simulink model "sampleModel1865"  (R2023a)
settings: Solver=VariableStepAuto  StartTime=0.0  StopTime=10.0  RelTol=1e-3
libraries: simulink x2, hdlsllib x2
settings Model: Creator=user1  LastModifiedBy=user1

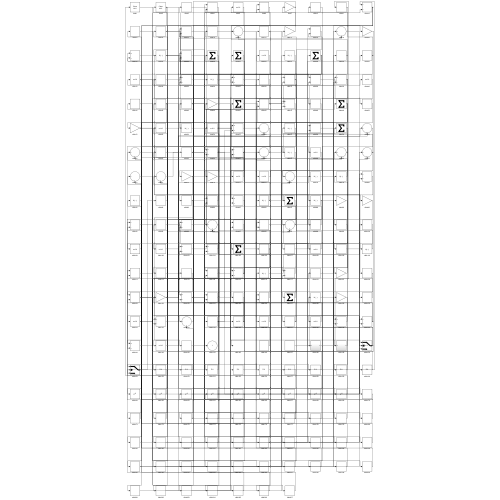
[thumbnail: Simulink's stored preview of the top-level diagram]
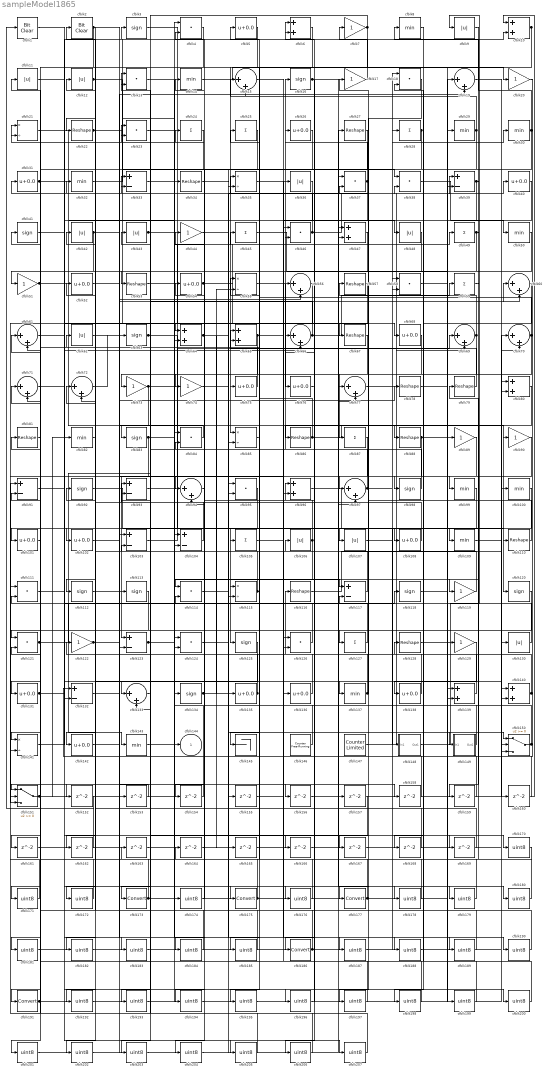
== system sampleModel1865 ==
  cfblk1 : simulink/Logic and Bit Operations/Bit Clear  iBit=0
      settings: LibrarySourceBlock=|
      | hdlsllib/Logic and Bit
      | Operations/Bit Clear
  cfblk{6,10,47,64..65,80,96,139..140} (9 alike) : Sum
  cfblk{8,14,29..30,32,50,82,99..100,109,137,143} (12 alike) : MinMax
  cfblk{5,26,31,40,52,54,68,75..76,101..102,108,131,135..136,138,142} (17 alike) : Bias  Bias=0.0  SaturateOnIntegerOverflow=off
  cfblk{33,39,91,93,103..104,117,123,132} (9 alike) : Sum  Inputs=+-
  cfblk{24..25,28,45,49,59,87,105,127} (9 alike) : Sum  Inputs=+
  cfblk{9,11..12,36,42..43,48,62,106..107,130} (11 alike) : Abs  SaturateOnIntegerOverflow=off
  cfblk{22,27,34,53,57,67,78..79,81,86,88,110,116,128} (14 alike) : Reshape
  cfblk{4,13,18,23,37..38,46,58,84,95,111,114,121,124,126} (15 alike) : DotProduct  OutDataTypeStr=Inherit: Inherit via internal rule
  cfblk{3,16,41,63,83,92,98,112..113,118,120,125,134} (13 alike) : Signum
  cfblk{21,35,55,85,115,141} (6 alike) : Product  Inputs=*/  RndMeth=Zero  SaturateOnIntegerOverflow=on
  cfblk{7,17,20,44,51,73..74,89..90,119,122,129} (12 alike) : Gain
  cfblk{15,19,56,60..61,66,69..72,77,94,97,133} (14 alike) : Sum  Inputs=|++
  cfblk145 : Terminator
  cfblk146 : hdlsllib/Sources/Counter Free-Running  NumBits=16  tsamp=-1
  cfblk147 : hdlsllib/Sources/Counter Limited  uplimit=7  tsamp=-1
  cfblk148 : Subsystem
      settings: LibrarySourceBlock=|
      | hdlsllib/Ports &
      | Subsystems/Subsystem
  cfblk149 : Subsystem
      settings: LibrarySourceBlock=|
      | hdlsllib/Ports &
      | Subsystems/Subsystem
  cfblk150 : Switch  SaturateOnIntegerOverflow=off  InputSameDT=off
  cfblk151 : Switch  SaturateOnIntegerOverflow=off  InputSameDT=off
  cfblk{152..169} (18 alike) : Delay  SampleTime=1
  cfblk{170..172,174,176,178..185,187..190,192..207} (33 alike) : DataTypeConversion  OutDataTypeStr=uint8  SaturateOnIntegerOverflow=off  RndMeth=Floor
  cfblk{173,175,177,186,191} (5 alike) : DataTypeConversion  SaturateOnIntegerOverflow=off  RndMeth=Floor
  cfblk2 : simulink/Logic and Bit Operations/Bit Clear  iBit=0
      settings: LibrarySourceBlock=|
      | hdlsllib/Logic and Bit
      | Operations/Bit Clear
  cfblk144 : Outport  VectorParamsAs1DForOutWhenUnconnected=off
  wires:
  cfblk17/1 -> cfblk7/1
  cfblk72/1 -> cfblk63/1
  cfblk89/1 -> cfblk123/1
  cfblk5/1 -> cfblk85/1
  cfblk151/1 -> cfblk82/1, cfblk104/2
  cfblk122/1 -> cfblk103/1, cfblk60/2
  cfblk9/1 -> cfblk114/1
  cfblk93/1 -> cfblk69/1
  cfblk103/1 -> cfblk49/1
  cfblk7/1 -> cfblk143/1, cfblk105/1
  cfblk83/1 -> cfblk172/1, cfblk176/1
  cfblk97/1 -> cfblk16/1, cfblk30/1
  cfblk11/1 -> cfblk175/1
  cfblk148/1(Out1) -> cfblk9/1
  cfblk73/1 -> cfblk123/2, cfblk60/1
  cfblk4/1 -> cfblk102/1
  cfblk140/1 -> cfblk116/1, cfblk93/2
  cfblk146/1 -> cfblk65/1
  cfblk53/1 -> cfblk45/1
  cfblk39/1 -> cfblk119/1, cfblk168/1
  cfblk12/1 -> cfblk38/1, cfblk34/1
  cfblk48/1 -> cfblk51/1
  cfblk107/1 -> cfblk28/1
  cfblk88/1 -> cfblk142/1, cfblk150/1
  cfblk92/1 -> cfblk125/1
  cfblk51/1 -> cfblk120/1, cfblk200/1
  cfblk63/1 -> cfblk110/1, cfblk10/2
  cfblk95/1 -> cfblk101/1
  cfblk37/1 -> cfblk133/1, cfblk26/1, cfblk77/1
  cfblk76/1 -> cfblk6/1
  cfblk108/1 -> cfblk93/1
  cfblk54/1 -> cfblk27/1, cfblk97/2
  cfblk33/1 -> cfblk144/1
  cfblk127/1 -> cfblk92/1
  cfblk16/1 -> cfblk178/1, cfblk206/1
  cfblk147/1 -> cfblk39/1
  cfblk115/1 -> cfblk55/1, cfblk4/2
  cfblk55/1 -> cfblk76/1
  cfblk137/1 -> cfblk17/1, cfblk122/1
  cfblk44/1 -> cfblk107/1
  cfblk124/1 -> cfblk37/2
  cfblk21/1 -> cfblk90/1
  cfblk20/1 -> cfblk132/1
  cfblk138/1 -> cfblk2/1
  cfblk1/1 -> cfblk68/1
  cfblk22/1 -> cfblk64/1, cfblk64/2, cfblk167/1
  cfblk84/1 -> cfblk83/1
  cfblk101/1 -> cfblk31/1
  cfblk10/1 -> cfblk121/1, cfblk53/1, cfblk139/2
  cfblk119/1 -> cfblk42/1
  cfblk3/1 -> cfblk135/1
  cfblk149/1(Out1) -> cfblk114/2
  cfblk31/1 -> cfblk134/1, cfblk66/2
  cfblk135/1 -> cfblk62/1, cfblk94/2
  cfblk57/1 -> cfblk141/1
  cfblk133/1 -> cfblk103/2
  cfblk106/1 -> cfblk115/1, cfblk21/1, cfblk145/1
  cfblk32/1 -> cfblk6/2
  cfblk68/1 -> cfblk86/1
  cfblk109/1 -> cfblk130/1
  cfblk110/1 -> cfblk33/1
  cfblk59/1 -> cfblk99/1
  cfblk70/1 -> cfblk25/1, cfblk73/1
  cfblk134/1 -> cfblk149/1(In1), cfblk55/2, cfblk204/1
  cfblk79/1 -> cfblk65/2
  cfblk25/1 -> cfblk74/1
  cfblk117/1 -> cfblk14/1
  cfblk46/1 -> cfblk29/1, cfblk38/2, cfblk21/2
  cfblk75/1 -> cfblk41/1
  cfblk8/1 -> cfblk98/1
  cfblk131/1 -> cfblk3/1, cfblk117/2
  cfblk41/1 -> cfblk140/2
  cfblk35/1 -> cfblk136/1
  cfblk36/1 -> cfblk132/2
  cfblk28/1 -> cfblk97/1, cfblk35/2, cfblk184/1
  cfblk139/1 -> cfblk23/1
  cfblk26/1 -> cfblk75/1
  cfblk60/1 -> cfblk138/1
  cfblk98/1 -> cfblk33/2
  cfblk86/1 -> cfblk88/1, cfblk35/1
  cfblk64/1 -> cfblk67/1, cfblk165/1
  cfblk118/1 -> cfblk19/1
  cfblk77/1 -> cfblk69/2
  cfblk116/1 -> cfblk70/2
  cfblk2/1 -> cfblk22/1, cfblk94/1, cfblk181/1
  cfblk45/1 -> cfblk139/1
  cfblk96/1 -> cfblk148/1(In1)
  cfblk42/1 -> cfblk112/1, cfblk96/2, cfblk171/1
  cfblk126/1 -> cfblk81/1
  cfblk82/1 -> cfblk32/1
  cfblk142/1 -> cfblk56/2
  cfblk105/1 -> cfblk36/1
  cfblk78/1 -> cfblk40/1
  cfblk29/1 -> cfblk131/1, cfblk15/2
  cfblk121/1 -> cfblk150/2, cfblk77/2, cfblk207/1
  cfblk30/1 -> cfblk8/1, cfblk192/1
  cfblk150/1 -> cfblk44/1, cfblk84/2
  cfblk104/1 -> cfblk72/2
  cfblk130/1 -> cfblk96/1
  cfblk47/1 -> cfblk191/1
  cfblk40/1 -> cfblk85/2
  cfblk15/1 -> cfblk48/1
  cfblk112/1 -> cfblk19/2
  cfblk18/1 -> cfblk177/1
  cfblk14/1 -> cfblk20/1
  cfblk56/1 -> cfblk151/3
  cfblk49/1 -> cfblk109/1, cfblk127/1, cfblk126/2
  cfblk38/1 -> cfblk50/1
  cfblk132/1 -> cfblk78/1
  cfblk87/1 -> cfblk141/2
  cfblk23/1 -> cfblk137/1
  cfblk136/1 -> cfblk54/1
  cfblk141/1 -> cfblk118/1
  cfblk123/1 -> cfblk179/1, cfblk190/1
  cfblk24/1 -> cfblk173/1
  cfblk65/1 -> cfblk115/2, cfblk188/1
  cfblk43/1 -> cfblk46/2, cfblk117/1
  cfblk66/1 -> cfblk59/1, cfblk13/1
  cfblk13/1 -> cfblk108/1
  cfblk69/1 -> cfblk57/1, cfblk87/1
  cfblk80/1 -> cfblk186/1
  cfblk6/1 -> cfblk152/1
  cfblk152/1 -> cfblk1/1
  cfblk62/1 -> cfblk153/1
  cfblk153/1 -> cfblk151/1
  cfblk94/1 -> cfblk154/1
  cfblk154/1 -> cfblk104/1
  cfblk155/1 -> cfblk56/1
  cfblk114/1 -> cfblk156/1
  cfblk156/1 -> cfblk10/1
  cfblk102/1 -> cfblk158/1
  cfblk158/1 -> cfblk72/1
  cfblk90/1 -> cfblk159/1
  cfblk159/1 -> cfblk15/1
  cfblk19/1 -> cfblk160/1
  cfblk160/1 -> cfblk66/1
  cfblk81/1 -> cfblk161/1
  cfblk161/1 -> cfblk46/1
  cfblk50/1 -> cfblk162/1
  cfblk162/1 -> cfblk151/2
  cfblk163/1 -> cfblk37/1
  cfblk164/1 -> cfblk140/1
  cfblk67/1 -> cfblk166/1
  cfblk166/1 -> cfblk70/1
  cfblk167/1 -> cfblk150/3
  cfblk168/1 -> cfblk23/2
  cfblk34/1 -> cfblk169/1
  cfblk169/1 -> cfblk12/1
  cfblk111/1 -> cfblk170/1
  cfblk170/1 -> cfblk164/1
  cfblk171/1 -> cfblk111/1
  cfblk172/1 -> cfblk111/2
  cfblk173/1 -> cfblk39/2, cfblk121/2
  cfblk143/1 -> cfblk174/1
  cfblk174/1 -> cfblk24/1
  cfblk175/1 -> cfblk163/1, cfblk13/2
  cfblk176/1 -> cfblk11/1
  cfblk177/1 -> cfblk5/1, cfblk133/2
  cfblk178/1 -> cfblk18/1
  cfblk179/1 -> cfblk18/2
  cfblk58/1 -> cfblk180/1
  cfblk180/1 -> cfblk79/1
  cfblk181/1 -> cfblk58/1
  cfblk125/1 -> cfblk182/1
  cfblk182/1 -> cfblk58/2
  cfblk61/1 -> cfblk183/1
  cfblk183/1 -> cfblk124/1
  cfblk184/1 -> cfblk61/1
  cfblk165/1 -> cfblk185/1
  cfblk185/1 -> cfblk61/2
  cfblk186/1 -> cfblk129/1, cfblk4/1
  cfblk74/1 -> cfblk187/1
  cfblk187/1 -> cfblk80/1
  cfblk188/1 -> cfblk80/2
  cfblk52/1 -> cfblk189/1
  cfblk189/1 -> cfblk84/1
  cfblk190/1 -> cfblk52/1
  cfblk191/1 -> cfblk124/2, cfblk89/1
  cfblk192/1 -> cfblk47/1
  cfblk27/1 -> cfblk193/1
  cfblk193/1 -> cfblk47/2
  cfblk100/1 -> cfblk194/1
  cfblk194/1 -> cfblk155/1
  cfblk85/1 -> cfblk195/1
  cfblk195/1 -> cfblk100/1
  cfblk71/1 -> cfblk196/1
  cfblk196/1 -> cfblk106/1
  cfblk99/1 -> cfblk197/1
  cfblk197/1 -> cfblk71/1
  cfblk129/1 -> cfblk198/1
  cfblk198/1 -> cfblk71/2
  cfblk128/1 -> cfblk199/1
  cfblk199/1 -> cfblk126/1
  cfblk200/1 -> cfblk128/1
  cfblk113/1 -> cfblk201/1
  cfblk201/1 -> cfblk95/1
  cfblk120/1 -> cfblk202/1
  cfblk202/1 -> cfblk113/1
  cfblk157/1 -> cfblk203/1
  cfblk203/1 -> cfblk95/2
  cfblk204/1 -> cfblk157/1
  cfblk91/1 -> cfblk205/1
  cfblk205/1 -> cfblk43/1
  cfblk206/1 -> cfblk91/1
  cfblk207/1 -> cfblk91/2

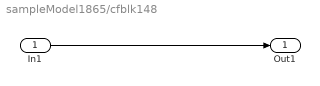
== system sampleModel1865/cfblk148 ==
  In1 : Inport
  Out1 : Outport
  wires:
  In1/1 -> Out1/1

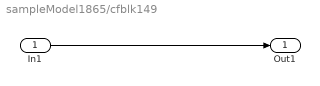
== system sampleModel1865/cfblk149 ==
  In1 : Inport
  Out1 : Outport
  wires:
  In1/1 -> Out1/1
